simulink model "function_demo"  (Simulink 6.3)
settings: Solver=ode45  StartTime=0.0  StopTime=10.0  RelTol=1e-3
settings Model: LastModifiedBy=Ms1

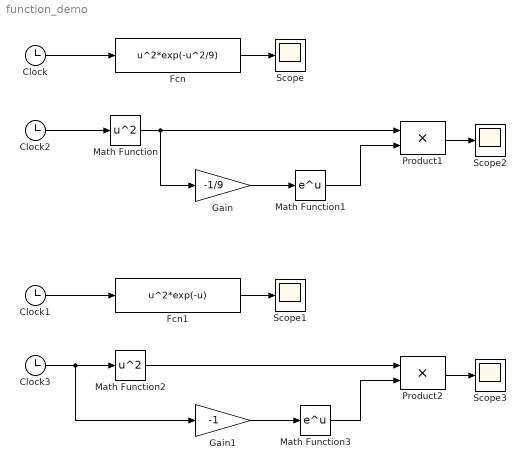
== system function_demo ==
  Clock{,1..3} (4 alike) : Clock
      settings: Decimation=10
  Fcn : Fcn  Expr=u^2*exp(-u^2/9)
  Fcn1 : Fcn  Expr=u^2*exp(-u)
  Gain : Gain  Gain=-1/9  SaturateOnIntegerOverflow=on
  Gain1 : Gain  Gain=-1  SaturateOnIntegerOverflow=on
  Math Function : Math  Operator=square  SaturateOnIntegerOverflow=on
  Math Function1 : Math  SaturateOnIntegerOverflow=on
  Math Function2 : Math  Operator=square  SaturateOnIntegerOverflow=on
  Math Function3 : Math  SaturateOnIntegerOverflow=on
  Product1 : Product  SaturateOnIntegerOverflow=on  InputSameDT=on
  Product2 : Product  SaturateOnIntegerOverflow=on  InputSameDT=on
  Scope{,1..3} (4 alike) : Scope
      Scope2 settings: SaveName=ScopeData2
      Scope3 settings: SaveName=ScopeData3
  wires:
  Clock/1 -> Fcn/1
  Fcn/1 -> Scope/1
  Clock1/1 -> Fcn1/1
  Fcn1/1 -> Scope1/1
  Clock2/1 -> Math Function/1
  Math Function/1 -> Gain/1, Product1/1
  Math Function1/1 -> Product1/2
  Product1/1 -> Scope2/1
  Gain/1 -> Math Function1/1
  Clock3/1 -> Math Function2/1, Gain1/1
  Math Function2/1 -> Product2/1
  Math Function3/1 -> Product2/2
  Product2/1 -> Scope3/1
  Gain1/1 -> Math Function3/1
